simulink model "Lab3"  (R2019b)
settings: Solver=VariableStepAuto  StartTime=0.0  StopTime=100  RelTol=1e-3
settings Model: Creator=Егор  LastModifiedBy=vak90
settings SolverCC: AlgebraicLoopSolver=LineSearch
settings DataIOCC: ReturnWorkspaceOutputs=off
settings DebuggingCC: ArithmeticOperatorsInVariantConditions=warning
settings SFSimCC: SimUseLocalCustomCode=off  CustomCodeUndefinedFunction=UseInterfaceOnly
settings RTWCC: RTWUseLocalCustomCode=off

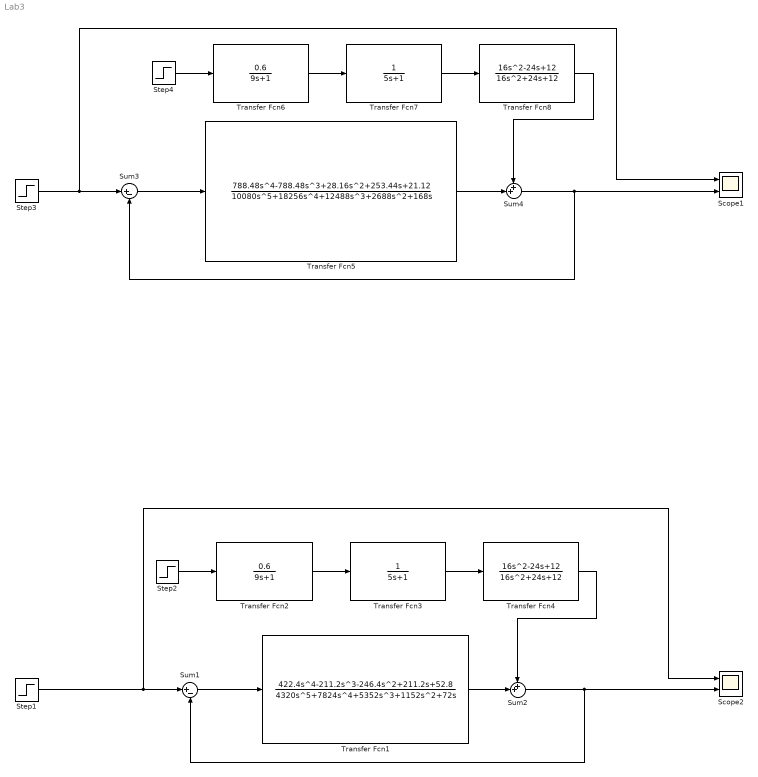
== system Lab3 ==
  Scope1 : Scope  NumInputPorts=2
  Scope2 : Scope  NumInputPorts=2
  Step1 : Step  SampleTime=0
  Step2 : Step  SampleTime=0
  Step3 : Step  Time=5  SampleTime=0
  Step4 : Step  SampleTime=0
  Sum1 : Sum  Inputs=|+-
  Sum2 : Sum  Inputs=++|
  Sum3 : Sum  Inputs=|+-
  Sum4 : Sum  Inputs=++|
  Transfer Fcn1 : TransferFcn  Numerator=[422.4 -211.2 -246.4 211.2 52.8]  Denominator=[4320 7824 5352 1152 72 0]
  Transfer Fcn2 : TransferFcn  Numerator=[0.6]  Denominator=[9 1]
  Transfer Fcn3 : TransferFcn  Denominator=[5 1]
  Transfer Fcn4 : TransferFcn  Numerator=[16 -24 12]  Denominator=[16 24 12]
  Transfer Fcn5 : TransferFcn  Numerator=[788.48 -788.48 28.16 253.44 21.12]  Denominator=[10080 18256 12488 2688 168 0]
  Transfer Fcn6 : TransferFcn  Numerator=[0.6]  Denominator=[9 1]
  Transfer Fcn7 : TransferFcn  Denominator=[5 1]
  Transfer Fcn8 : TransferFcn  Numerator=[16 -24 12]  Denominator=[16 24 12]
  wires:
  Step1/1 -> Scope2/1, Sum1/1
  Sum1/1 -> Transfer Fcn1/1
  Transfer Fcn1/1 -> Sum2/2
  Sum2/1 -> Sum1/2, Scope2/2
  Transfer Fcn2/1 -> Transfer Fcn3/1
  Transfer Fcn3/1 -> Transfer Fcn4/1
  Transfer Fcn4/1 -> Sum2/1
  Step2/1 -> Transfer Fcn2/1
  Sum3/1 -> Transfer Fcn5/1
  Step3/1 -> Sum3/1, Scope1/1
  Transfer Fcn5/1 -> Sum4/2
  Sum4/1 -> Sum3/2, Scope1/2
  Step4/1 -> Transfer Fcn6/1
  Transfer Fcn7/1 -> Transfer Fcn8/1
  Transfer Fcn6/1 -> Transfer Fcn7/1
  Transfer Fcn8/1 -> Sum4/1
